simulink model "KerstingThreePhase"  (R2020a)
settings: Solver=ode45  StartTime=0.0  StopTime=2  RelTol=1e-3  EnableMultiTasking=on
undefined symbols (not defined in the file): Ac, Bc, Cc, Dc, j
libraries: powerlib x14, powerlib_meascontrol x9, simulink_extras x6
settings Model: Creator=Matus  LastModifiedBy=VaioPC
settings DataIOCC: LimitDataPoints=on  SaveFormat=Array  ReturnWorkspaceOutputs=off
settings OptimizationCC: LifeSpan=inf
settings DebuggingCC: UnderspecifiedInitializationDetection=Classic  MergeDetectMultiDrivingBlocksExec=none  StateNameClashWarn=warning  SFUnexpectedBacktrackingDiag=warning  SFNoUnconditionalDefaultTransitionDiag=warning  SFExecutionAtInitializationDiag=none  ArithmeticOperatorsInVariantConditions=warning
settings HardwareCC: ProdBitPerPointer=32  ProdBitPerSizeT=32  ProdBitPerPtrDiffT=32  ProdLargestAtomicFloat=None  ProdIntDivRoundTo=Undefined  ProdEndianess=Unspecified  ProdWordSize=32  ProdHWDeviceType=32-bit Generic
settings ModelReferenceCC: PropagateSignalLabelsOutOfModel=off
settings SFSimCC: SimUseLocalCustomCode=off  CustomCodeUndefinedFunction=UseInterfaceOnly
settings RTWCC: RTWUseLocalCustomCode=off
settings CodeAppCC: StateflowObjectComments=on
settings GRTTargetCC: TargetLangStandard=C89/C90 (ANSI)
settings ConfigComp: CovMetricSettings=dw  CovHtmlReporting=on  CovSaveCumulativeToWorkspaceVar=on  CovSaveSingleToWorkspaceVar=on  CovExternalEMLEnable=off
settings SimscapeCC: SimscapeNormalizeSystem=off

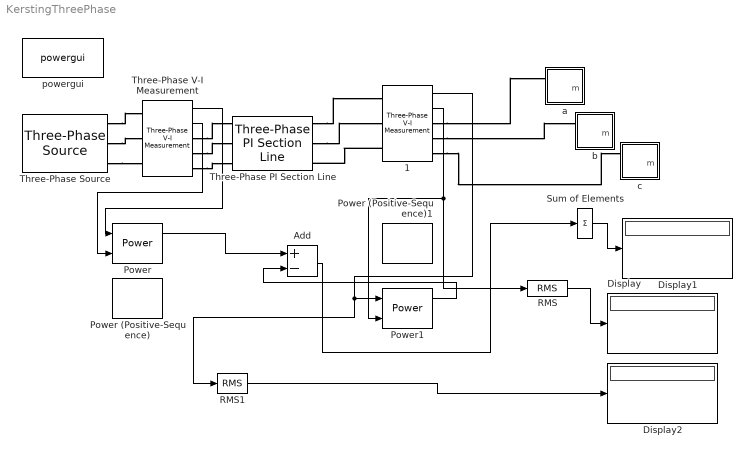
== system KerstingThreePhase ==
  1 : powerlib/Measurements/Three-Phase V-I Measurement  VoltageMeasurement=phase-to-ground  SetLabelV=off  LabelV=Vabc  Vpu=off  VpuLL=off  CurrentMeasurement=yes  SetLabelI=off  LabelI=Iabc  Ipu=off  Pbase=100e6  Vbase=500e3  OutputType=Complex  PhasorSimulation=off  PSBequivalent=0
  Add : Sum  Inputs=+-
  Display : Display
  Display1 : Display
  Display2 : Display
  Power : powerlib_meascontrol/Measurements/Power  Freq=60  Vinit=[1, 0]  Iinit=[1, 0]  Ts=0
  Power (Positive-Sequence) : powerlib_meascontrol/Measurements/Power (Positive-Sequence)  Freq=60  Vinit=[0, 0]  Iinit=[0, 0]  Ts=0
      settings: SourceProductBaseCode=PS
  Power (Positive-Sequence)1 : powerlib_meascontrol/Measurements/Power (Positive-Sequence)  Freq=60  Vinit=[0, 0]  Iinit=[0, 0]  Ts=0
      settings: SourceProductBaseCode=PS
  Power1 : powerlib_meascontrol/Measurements/Power  Freq=60  Vinit=[1, 0]  Iinit=[1, 0]  Ts=0
  RMS : powerlib_meascontrol/Measurements/RMS  TrueRMS=on  Freq=60  RMSInit=120  Ts=0
  RMS1 : powerlib_meascontrol/Measurements/RMS  TrueRMS=on  Freq=60  RMSInit=120  Ts=0
  Sum of Elements : Sum  Inputs=+
  Three-Phase PI Section Line : powerlib/Elements/Three-Phase PI Section Line  LConnTagsString=a|b|c  RConnTagsString=A|B|C  Frequency=60  Resistances=[ 0.1902 0.4807]  Inductances="[ 1.0336e-3  3.1935e-3]"  Capacitances=[12.74e-9 7.751e-9]  Length=1.8182
  Three-Phase V-I Measurement : powerlib/Measurements/Three-Phase V-I Measurement  VoltageMeasurement=phase-to-ground  SetLabelV=off  LabelV=Vabc  Vpu=off  VpuLL=off  CurrentMeasurement=yes  SetLabelI=off  LabelI=Iabc  Ipu=off  Pbase=100e6  Vbase=500e3  OutputType=Complex  PhasorSimulation=off  PSBequivalent=0
  Three-Phase Source : powerlib/Electrical Sources/Three-Phase Source  InternalConnection=Yg  VoltagePhases=off  Voltage=12470  PhaseAngle=0  Voltage_phases=[25e3 25e3 25e3]/sqrt(3)  PhaseAngles_phases=[0 -120 +120]  Frequency=60  NonIdealSource=on  SpecifyImpedance=on  Resistance=0.8929  Inductance=16.58e-3  ShortCircuitLevel=500e6  BaseVoltage=12470  XRratio=3  BusType=swing  Pref=0  Qref=0  Prefabc=[10e3, 10e3, 10e3]  Qrefabc=[0, 0, 0]  Qmin=-inf  Qmax=inf
  a : Subsystem  DialogController=POWERSYS.PowerSysDialog  mask(Single-Phase Dynamic Load){NominalVoltage=[ 7.1999e3 60 ], ActiveReactivePowers=[2.7e6 1.3077e6], PositiveSequence=[1 0], ExternalControl=off, NpNq=[0 0], TimeConstants=[0  0  0  0], MinimumVoltage=0.7, LoadFlowParameters=[4,0,0,0,0]}
      mask prompts: NominalVoltage "Nominal voltage and frequency  [Vn(Vrms) fn(Hz)]:"; ActiveReactivePowers "Active and reactive power at initial voltage [Po(W) Qo(var)]:"; PositiveSequence "Initial voltage Vo [Mag(pu) Phase (deg.)]:"; ExternalControl "External control of PQ"; NpNq "Parameters [ np  nq ]:"; TimeConstants "Time constants [Tp1 Tp2 Tq1 Tq2]  (s):"; MinimumVoltage "Minimum voltage Vmin (pu):"; LoadFlowParameters "Load Flow parameters"
      mask help:
      | Implements a single-phase dynamic load. Active  power P and reactive
      | power Q absorbed by the load vary as function of voltage V  according to the
      | following equations:
      |
      |   If V>Vmin, P and Q vary as follows:
      |        P = Po * (V/Vo)^np * (1+Tp1.s)/(1+Tp2.s)
      |        Q = Qo * (V/Vo)^nq * (1+Tq1.s)/(1+Tq2.s)
      |   if V<Vmin
      |      Same equations with np=nq=2 (constant impedance load)
      mask init:
      | block = gcb;
      | Ts = 50e-6;
      | %
      | Vnom=NominalVoltage(1); 
      | fnom=NominalVoltage(2);
      | P0=ActiveReactivePowers(1);
      | Q0=ActiveReactivePowers(2);
      | Mag_V0=PositiveSequence(1); 
      | Pha_V0=PositiveSequence(2);
      | V0_d=Mag_V0*cos(Pha_V0*pi/180);
      | V0_q=Mag_V0*sin(Pha_V0*pi/180);
      | np=NpNq(1);
      | nq=NpNq(2);
      | Tp1=TimeConstants(1); 
      | Tp2=TimeConstants(2); 
      | Tq1=TimeConstants(3); 
      | Tq2=TimeConstants(4);
      | Vbase=Vnom/sqrt(3)*sqrt(2);
      | % initial value of positive-sequence current I1
      | I1_init=(P0-j*Q0)/((V0_d-j*V0_q)*Vnom)/sqrt(3)*sqrt(2);
      | Mag_ia=abs(I1_init);
      | Phase_ia=angle(I1_init)*180/pi;
      | %
      | Vmin=MinimumVoltage;
      | PQext=ExternalControl;
      | a=exp(j*2*pi/3);
      | power_initmask();
      mask Help: helpview(psbhelp)
      mask Callback ExternalControl: powericon('ThreePhaseDynamicLoadCback',gcb);
      mask Display:
      | plot(-45,-45,45,45,[0,9,18,24,29,30,29,24,18,9,0,-9,-18,-24,-29,-30,-29,-24,-18,-9,0]*.9,[30,29,24,18,9,0,-9,-18,-24,-29,-30,-29,-24,-18,-9,0,9,18,24,29,30]*.9)
      | plot([0,0,10,0,-10,0]*1.1,[15,-5,-5,-15,-5,-5]*1.1)
  b : Subsystem  DialogController=POWERSYS.PowerSysDialog  mask(Single-Phase Dynamic Load){NominalVoltage=[ 7.1999e3 60 ], ActiveReactivePowers=[3.3250e6 1.0929e6], PositiveSequence=[1 0], ExternalControl=off, NpNq=[0 0], TimeConstants=[0  0  0  0], MinimumVoltage=0.7, LoadFlowParameters=[4,0,0,0,0]}
      mask prompts: NominalVoltage "Nominal voltage and frequency  [Vn(Vrms) fn(Hz)]:"; ActiveReactivePowers "Active and reactive power at initial voltage [Po(W) Qo(var)]:"; PositiveSequence "Initial voltage Vo [Mag(pu) Phase (deg.)]:"; ExternalControl "External control of PQ"; NpNq "Parameters [ np  nq ]:"; TimeConstants "Time constants [Tp1 Tp2 Tq1 Tq2]  (s):"; MinimumVoltage "Minimum voltage Vmin (pu):"; LoadFlowParameters "Load Flow parameters"
      mask help:
      | Implements a single-phase dynamic load. Active  power P and reactive
      | power Q absorbed by the load vary as function of voltage V  according to the
      | following equations:
      |
      |   If V>Vmin, P and Q vary as follows:
      |        P = Po * (V/Vo)^np * (1+Tp1.s)/(1+Tp2.s)
      |        Q = Qo * (V/Vo)^nq * (1+Tq1.s)/(1+Tq2.s)
      |   if V<Vmin
      |      Same equations with np=nq=2 (constant impedance load)
      mask init: same as KerstingThreePhase/a
      mask Help: helpview(psbhelp)
      mask Callback ExternalControl: powericon('ThreePhaseDynamicLoadCback',gcb);
      mask Display:
      | plot(-45,-45,45,45,[0,9,18,24,29,30,29,24,18,9,0,-9,-18,-24,-29,-30,-29,-24,-18,-9,0]*.9,[30,29,24,18,9,0,-9,-18,-24,-29,-30,-29,-24,-18,-9,0,9,18,24,29,30]*.9)
      | plot([0,0,10,0,-10,0]*1.1,[15,-5,-5,-15,-5,-5]*1.1)
  c : Subsystem  DialogController=POWERSYS.PowerSysDialog  mask(Single-Phase Dynamic Load){NominalVoltage=[ 7.1999e3 60 ], ActiveReactivePowers=[2.1250e6 1.3170e6], PositiveSequence=[1 0], ExternalControl=off, NpNq=[0 0], TimeConstants=[0  0  0  0], MinimumVoltage=0.7, LoadFlowParameters=[4,0,0,0,0]}
      mask prompts: NominalVoltage "Nominal voltage and frequency  [Vn(Vrms) fn(Hz)]:"; ActiveReactivePowers "Active and reactive power at initial voltage [Po(W) Qo(var)]:"; PositiveSequence "Initial voltage Vo [Mag(pu) Phase (deg.)]:"; ExternalControl "External control of PQ"; NpNq "Parameters [ np  nq ]:"; TimeConstants "Time constants [Tp1 Tp2 Tq1 Tq2]  (s):"; MinimumVoltage "Minimum voltage Vmin (pu):"; LoadFlowParameters "Load Flow parameters"
      mask help:
      | Implements a single-phase dynamic load. Active  power P and reactive
      | power Q absorbed by the load vary as function of voltage V  according to the
      | following equations:
      |
      |   If V>Vmin, P and Q vary as follows:
      |        P = Po * (V/Vo)^np * (1+Tp1.s)/(1+Tp2.s)
      |        Q = Qo * (V/Vo)^nq * (1+Tq1.s)/(1+Tq2.s)
      |   if V<Vmin
      |      Same equations with np=nq=2 (constant impedance load)
      mask init: same as KerstingThreePhase/a
      mask Help: helpview(psbhelp)
      mask Callback ExternalControl: powericon('ThreePhaseDynamicLoadCback',gcb);
      mask Display:
      | plot(-45,-45,45,45,[0,9,18,24,29,30,29,24,18,9,0,-9,-18,-24,-29,-30,-29,-24,-18,-9,0]*.9,[30,29,24,18,9,0,-9,-18,-24,-29,-30,-29,-24,-18,-9,0,9,18,24,29,30]*.9)
      | plot([0,0,10,0,-10,0]*1.1,[15,-5,-5,-15,-5,-5]*1.1)
  powergui : powerlib/powergui  Priority=1  SimulationMode=Discrete  SampleTime=50e-6  frequency=60  Iterations=50  frequencyindice=60  Pbase=100e6  ErrMax=1e-4  UnitsV=kV  UnitsW=MW  buscounter=0  FunctionMessages=off  echomessages=off  EnableUseOfTLC=off  CurrentSourceSwitches=off  DisableSnubberDevices=off  DisableRonSwitches=off  DisableVfSwitches=off  DisplayEquations=off  AutomaticDiscreteSolvers=off  SolverType=Tustin/Backward Euler (TBE)  Interpol=off  ExternalGateDelay=off  methode=off  Ts=100  x0status=blocks  SPID=on  SwTol=0  HookPort=off  NonlinearTolerance=1e-4  nMaxIteration=100  ContinueOnMaxIteration=off  RestoreLinks=warning  ResistiveCurrentMeasurement=off  Frange=[0:2:500]  Ylog=off  Xlog=on  ShowGrid=off  save=off  variable=ZData  structure=0  ZoomFFT=off  StartTime=0.0  cycles=1  DisplayStyle=1  fundamental=60  FreqAxis=off  MaxFrequency=1000  frequencyindicesteady=1  RmsSteady=2  display=off
  wires:
  Three-Phase V-I Measurement/2 -> Power/2
  Three-Phase V-I Measurement/1 -> Power/1
  1/1 -> Power1/1, RMS1/1
  1/2 -> Power1/2, RMS/1
  RMS/1 -> Display/1
  RMS1/1 -> Display2/1
  Add/1 -> Sum of Elements/1
  Power/1 -> Add/1
  Power1/1 -> Add/2
  Sum of Elements/1 -> Display1/1
  connections:
  Three-Phase Source/RConn1 -- Three-Phase V-I Measurement/LConn1
  Three-Phase Source/RConn2 -- Three-Phase V-I Measurement/LConn2
  Three-Phase Source/RConn3 -- Three-Phase V-I Measurement/LConn3
  1/LConn3 -- Three-Phase PI Section Line/RConn3
  Three-Phase PI Section Line/RConn2 -- 1/LConn2
  Three-Phase PI Section Line/RConn1 -- 1/LConn1
  Three-Phase V-I Measurement/RConn1 -- Three-Phase PI Section Line/LConn1
  Three-Phase V-I Measurement/RConn2 -- Three-Phase PI Section Line/LConn2
  Three-Phase V-I Measurement/RConn3 -- Three-Phase PI Section Line/LConn3
  1/RConn1 -- a/LConn1
  1/RConn2 -- b/LConn1
  1/RConn3 -- c/LConn1

== system KerstingThreePhase/a ==
  Controlled Current Source : powerlib/Electrical Sources/Controlled Current Source  Initialize=on  Source_Type=AC  Amplitude=0  Phase=0  Frequency=0  Measurements=None
  Gain : Gain  Gain=-1
  Ground1 : powerlib/Elements/Ground  LConnTagsString=a
  Measurement list : Subsystem
  PQ : Ground
  Voltage Measurement1 : powerlib/Measurements/Voltage Measurement  PhasorSimulation=off  OutputType=Complex  PSBequivalent=0
  model : Subsystem
  a : PMIOPort  Tag=PMCPort  Side=Left
  b : PMIOPort  Tag=PMCPort  Port=2  Side=Left
  m : Outport  InitialOutput=[0,0,0]  VectorParamsAs1DForOutWhenUnconnected=off
  wires:
  Gain/1 -> Controlled Current Source/1
  Measurement list/1(Out1) -> m/1
  model/1(i) -> Gain/1
  Voltage Measurement1/1 -> model/1(v)
  PQ/1 -> model/2(PQ)
  model/2(m) -> Measurement list/1(In1)
  connections:
  Controlled Current Source/LConn1 -- Ground1/LConn1 -- b/RConn1 -- Voltage Measurement1/LConn2
  Controlled Current Source/RConn1 -- a/RConn1 -- Voltage Measurement1/LConn1

== system KerstingThreePhase/b ==
  Controlled Current Source : powerlib/Electrical Sources/Controlled Current Source  Initialize=on  Source_Type=AC  Amplitude=0  Phase=0  Frequency=0  Measurements=None
  Gain : Gain  Gain=-1
  Ground1 : powerlib/Elements/Ground  LConnTagsString=a
  Measurement list : Subsystem
  PQ : Ground
  Voltage Measurement1 : powerlib/Measurements/Voltage Measurement  PhasorSimulation=off  OutputType=Complex  PSBequivalent=0
  model : Subsystem
  a : PMIOPort  Tag=PMCPort  Side=Left
  b : PMIOPort  Tag=PMCPort  Port=2  Side=Left
  m : Outport  InitialOutput=[0,0,0]  VectorParamsAs1DForOutWhenUnconnected=off
  wires:
  Gain/1 -> Controlled Current Source/1
  Measurement list/1(Out1) -> m/1
  model/1(i) -> Gain/1
  Voltage Measurement1/1 -> model/1(v)
  PQ/1 -> model/2(PQ)
  model/2(m) -> Measurement list/1(In1)
  connections:
  Controlled Current Source/LConn1 -- Voltage Measurement1/LConn2 -- Ground1/LConn1 -- b/RConn1
  Controlled Current Source/RConn1 -- a/RConn1 -- Voltage Measurement1/LConn1

== system KerstingThreePhase/c ==
  Controlled Current Source : powerlib/Electrical Sources/Controlled Current Source  Initialize=on  Source_Type=AC  Amplitude=0  Phase=0  Frequency=0  Measurements=None
  Gain : Gain  Gain=-1
  Ground1 : powerlib/Elements/Ground  LConnTagsString=a
  Measurement list : Subsystem
  PQ : Ground
  Voltage Measurement1 : powerlib/Measurements/Voltage Measurement  PhasorSimulation=off  OutputType=Complex  PSBequivalent=0
  model : Subsystem
  a : PMIOPort  Tag=PMCPort  Side=Left
  b : PMIOPort  Tag=PMCPort  Port=2  Side=Left
  m : Outport  InitialOutput=[0,0,0]  VectorParamsAs1DForOutWhenUnconnected=off
  wires:
  Gain/1 -> Controlled Current Source/1
  Measurement list/1(Out1) -> m/1
  model/1(i) -> Gain/1
  Voltage Measurement1/1 -> model/1(v)
  PQ/1 -> model/2(PQ)
  model/2(m) -> Measurement list/1(In1)
  connections:
  Controlled Current Source/LConn1 -- Voltage Measurement1/LConn2 -- Ground1/LConn1 -- b/RConn1
  Controlled Current Source/RConn1 -- a/RConn1 -- Voltage Measurement1/LConn1

== system KerstingThreePhase/a/Measurement list ==
  In1 : Inport
  Bus Creator1 : BusCreator  Inputs=3
  Demux : Demux  Outputs=[1,1,1]
  Out1 : Outport  VectorParamsAs1DForOutWhenUnconnected=off
  wires:
  In1/1 -> Demux/1
  Bus Creator1/1 -> Out1/1
  Demux/2 -> Bus Creator1/2  "Active power P (W)"
  Demux/1 -> Bus Creator1/1  "Positive-sequence voltage V (pu)"
  Demux/3 -> Bus Creator1/3  "Reactive power Q (var)"

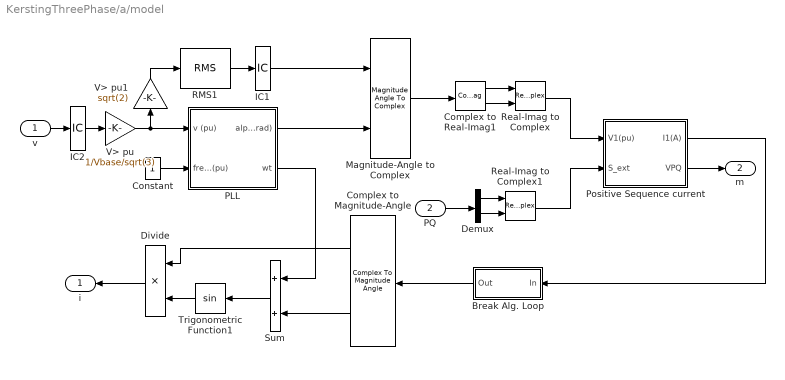
== system KerstingThreePhase/a/model ==
  v : Inport
  PQ : Inport  Port=2
  Break Alg. Loop : Subsystem
  Complex to Magnitude-Angle : ComplexToMagnitudeAngle
  Complex to Real-Imag1 : ComplexToRealImag
  Constant : Constant
  Demux : Demux  Outputs=2
      settings: DisplayOption=none
  Divide : Product  Inputs=**
  IC1 : InitialCondition
  IC2 : InitialCondition
  Magnitude-Angle to Complex : MagnitudeAngleToComplex
  PLL : Subsystem  mask{freq=fnom}
      mask prompts: freq "Initial frequency (Hz)"
  Positive Sequence current : Subsystem
  RMS1 : powerlib_meascontrol/Measurements/RMS  TrueRMS=on  Freq=fnom  RMSInit=1  Ts=0
  Real-Imag to Complex : RealImagToComplex
  Real-Imag to Complex1 : RealImagToComplex
  Sum : Sum
  Trigonometric Function1 : Trigonometry
  V> pu : Gain  Gain=1/Vbase/sqrt(3)  SaturateOnIntegerOverflow=on  OutDataTypeStr=Inherit: Same as input  ParamDataTypeStr=Inherit: Same as input
  V> pu1 : Gain  Gain=sqrt(2)  SaturateOnIntegerOverflow=on  OutDataTypeStr=Inherit: Same as input  ParamDataTypeStr=Inherit: Same as input
  i : Outport  VectorParamsAs1DForOutWhenUnconnected=off
  m : Outport  Port=2  VectorParamsAs1DForOutWhenUnconnected=off
  wires:
  IC2/1 -> V> pu/1
  V> pu1/1 -> RMS1/1
  IC1/1 -> Magnitude-Angle to Complex/1
  RMS1/1 -> IC1/1
  Break Alg. Loop/1(Out) -> Complex to Magnitude-Angle/1
  Divide/1 -> i/1
  Complex to Magnitude-Angle/1 -> Divide/1
  Trigonometric Function1/1 -> Divide/2
  Sum/1 -> Trigonometric Function1/1
  PLL/2(wt) -> Sum/1
  Complex to Magnitude-Angle/2 -> Sum/2
  PLL/1(alpha (rad)) -> Magnitude-Angle to Complex/2
  Constant/1 -> PLL/2(freq (pu))
  Magnitude-Angle to Complex/1 -> Complex to Real-Imag1/1
  Complex to Real-Imag1/2 -> Real-Imag to Complex/2
  Complex to Real-Imag1/1 -> Real-Imag to Complex/1
  v/1 -> IC2/1
  Positive Sequence current/2(VPQ) -> m/1
  Real-Imag to Complex1/1 -> Positive Sequence current/2(S_ext)
  Demux/2 -> Real-Imag to Complex1/2
  Demux/1 -> Real-Imag to Complex1/1
  PQ/1 -> Demux/1
  Positive Sequence current/1(I1(A)) -> Break Alg. Loop/1(In)
  Real-Imag to Complex/1 -> Positive Sequence current/1(V1(pu))
  V> pu/1 -> V> pu1/1, PLL/1(v (pu))

== system KerstingThreePhase/b/Measurement list ==
  In1 : Inport
  Bus Creator1 : BusCreator  Inputs=3
  Demux : Demux  Outputs=[1,1,1]
  Out1 : Outport  VectorParamsAs1DForOutWhenUnconnected=off
  wires:
  In1/1 -> Demux/1
  Bus Creator1/1 -> Out1/1
  Demux/2 -> Bus Creator1/2  "Active power P (W)"
  Demux/1 -> Bus Creator1/1  "Positive-sequence voltage V (pu)"
  Demux/3 -> Bus Creator1/3  "Reactive power Q (var)"

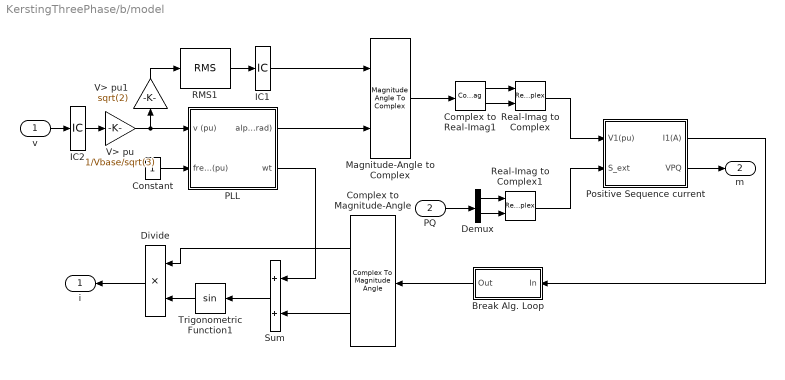
== system KerstingThreePhase/b/model ==
  v : Inport
  PQ : Inport  Port=2
  Break Alg. Loop : Subsystem
  Complex to Magnitude-Angle : ComplexToMagnitudeAngle
  Complex to Real-Imag1 : ComplexToRealImag
  Constant : Constant
  Demux : Demux  Outputs=2
      settings: DisplayOption=none
  Divide : Product  Inputs=**
  IC1 : InitialCondition
  IC2 : InitialCondition
  Magnitude-Angle to Complex : MagnitudeAngleToComplex
  PLL : Subsystem  mask{freq=fnom}
      mask prompts: freq "Initial frequency (Hz)"
  Positive Sequence current : Subsystem
  RMS1 : powerlib_meascontrol/Measurements/RMS  TrueRMS=on  Freq=fnom  RMSInit=1  Ts=0
  Real-Imag to Complex : RealImagToComplex
  Real-Imag to Complex1 : RealImagToComplex
  Sum : Sum
  Trigonometric Function1 : Trigonometry
  V> pu : Gain  Gain=1/Vbase/sqrt(3)  SaturateOnIntegerOverflow=on  OutDataTypeStr=Inherit: Same as input  ParamDataTypeStr=Inherit: Same as input
  V> pu1 : Gain  Gain=sqrt(2)  SaturateOnIntegerOverflow=on  OutDataTypeStr=Inherit: Same as input  ParamDataTypeStr=Inherit: Same as input
  i : Outport  VectorParamsAs1DForOutWhenUnconnected=off
  m : Outport  Port=2  VectorParamsAs1DForOutWhenUnconnected=off
  wires:
  IC2/1 -> V> pu/1
  V> pu1/1 -> RMS1/1
  IC1/1 -> Magnitude-Angle to Complex/1
  RMS1/1 -> IC1/1
  Break Alg. Loop/1(Out) -> Complex to Magnitude-Angle/1
  Divide/1 -> i/1
  Complex to Magnitude-Angle/1 -> Divide/1
  Trigonometric Function1/1 -> Divide/2
  Sum/1 -> Trigonometric Function1/1
  PLL/2(wt) -> Sum/1
  Complex to Magnitude-Angle/2 -> Sum/2
  PLL/1(alpha (rad)) -> Magnitude-Angle to Complex/2
  Constant/1 -> PLL/2(freq (pu))
  Magnitude-Angle to Complex/1 -> Complex to Real-Imag1/1
  Complex to Real-Imag1/2 -> Real-Imag to Complex/2
  Complex to Real-Imag1/1 -> Real-Imag to Complex/1
  v/1 -> IC2/1
  Positive Sequence current/2(VPQ) -> m/1
  Real-Imag to Complex1/1 -> Positive Sequence current/2(S_ext)
  Demux/2 -> Real-Imag to Complex1/2
  Demux/1 -> Real-Imag to Complex1/1
  PQ/1 -> Demux/1
  Positive Sequence current/1(I1(A)) -> Break Alg. Loop/1(In)
  Real-Imag to Complex/1 -> Positive Sequence current/1(V1(pu))
  V> pu/1 -> V> pu1/1, PLL/1(v (pu))

== system KerstingThreePhase/c/Measurement list ==
  In1 : Inport
  Bus Creator1 : BusCreator  Inputs=3
  Demux : Demux  Outputs=[1,1,1]
  Out1 : Outport  VectorParamsAs1DForOutWhenUnconnected=off
  wires:
  In1/1 -> Demux/1
  Bus Creator1/1 -> Out1/1
  Demux/2 -> Bus Creator1/2  "Active power P (W)"
  Demux/1 -> Bus Creator1/1  "Positive-sequence voltage V (pu)"
  Demux/3 -> Bus Creator1/3  "Reactive power Q (var)"

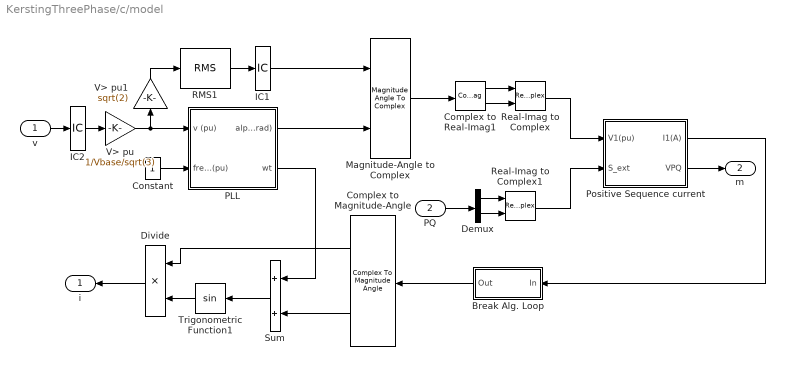
== system KerstingThreePhase/c/model ==
  v : Inport
  PQ : Inport  Port=2
  Break Alg. Loop : Subsystem
  Complex to Magnitude-Angle : ComplexToMagnitudeAngle
  Complex to Real-Imag1 : ComplexToRealImag
  Constant : Constant
  Demux : Demux  Outputs=2
      settings: DisplayOption=none
  Divide : Product  Inputs=**
  IC1 : InitialCondition
  IC2 : InitialCondition
  Magnitude-Angle to Complex : MagnitudeAngleToComplex
  PLL : Subsystem  mask{freq=fnom}
      mask prompts: freq "Initial frequency (Hz)"
  Positive Sequence current : Subsystem
  RMS1 : powerlib_meascontrol/Measurements/RMS  TrueRMS=on  Freq=fnom  RMSInit=1  Ts=0
  Real-Imag to Complex : RealImagToComplex
  Real-Imag to Complex1 : RealImagToComplex
  Sum : Sum
  Trigonometric Function1 : Trigonometry
  V> pu : Gain  Gain=1/Vbase/sqrt(3)  SaturateOnIntegerOverflow=on  OutDataTypeStr=Inherit: Same as input  ParamDataTypeStr=Inherit: Same as input
  V> pu1 : Gain  Gain=sqrt(2)  SaturateOnIntegerOverflow=on  OutDataTypeStr=Inherit: Same as input  ParamDataTypeStr=Inherit: Same as input
  i : Outport  VectorParamsAs1DForOutWhenUnconnected=off
  m : Outport  Port=2  VectorParamsAs1DForOutWhenUnconnected=off
  wires:
  IC2/1 -> V> pu/1
  V> pu1/1 -> RMS1/1
  IC1/1 -> Magnitude-Angle to Complex/1
  RMS1/1 -> IC1/1
  Break Alg. Loop/1(Out) -> Complex to Magnitude-Angle/1
  Divide/1 -> i/1
  Complex to Magnitude-Angle/1 -> Divide/1
  Trigonometric Function1/1 -> Divide/2
  Sum/1 -> Trigonometric Function1/1
  PLL/2(wt) -> Sum/1
  Complex to Magnitude-Angle/2 -> Sum/2
  PLL/1(alpha (rad)) -> Magnitude-Angle to Complex/2
  Constant/1 -> PLL/2(freq (pu))
  Magnitude-Angle to Complex/1 -> Complex to Real-Imag1/1
  Complex to Real-Imag1/2 -> Real-Imag to Complex/2
  Complex to Real-Imag1/1 -> Real-Imag to Complex/1
  v/1 -> IC2/1
  Positive Sequence current/2(VPQ) -> m/1
  Real-Imag to Complex1/1 -> Positive Sequence current/2(S_ext)
  Demux/2 -> Real-Imag to Complex1/2
  Demux/1 -> Real-Imag to Complex1/1
  PQ/1 -> Demux/1
  Positive Sequence current/1(I1(A)) -> Break Alg. Loop/1(In)
  Real-Imag to Complex/1 -> Positive Sequence current/1(V1(pu))
  V> pu/1 -> V> pu1/1, PLL/1(v (pu))

== system KerstingThreePhase/a/model/Break Alg. Loop ==
  In : Inport
  Complex to Real-Imag : ComplexToRealImag
  Real-Imag to Complex : RealImagToComplex
  imag : simulink_extras/Additional Linear/Transfer Fcn (with initial outputs)  N=[1]  D="[100e-6  1]"  Y0=imag(I1_init*exp(-j*Pha_V0*pi/180))  U0=imag(I1_init*exp(-j*Pha_V0*pi/180))
  real : simulink_extras/Additional Linear/Transfer Fcn (with initial outputs)  N=[1]  D="[100e-6  1]"  Y0=real(I1_init*exp(-j*Pha_V0*pi/180))  U0=real(I1_init*exp(-j*Pha_V0*pi/180))
  Out : Outport  VectorParamsAs1DForOutWhenUnconnected=off
  wires:
  In/1 -> Complex to Real-Imag/1
  Real-Imag to Complex/1 -> Out/1
  Complex to Real-Imag/1 -> real/1
  real/1 -> Real-Imag to Complex/1
  Complex to Real-Imag/2 -> imag/1
  imag/1 -> Real-Imag to Complex/2

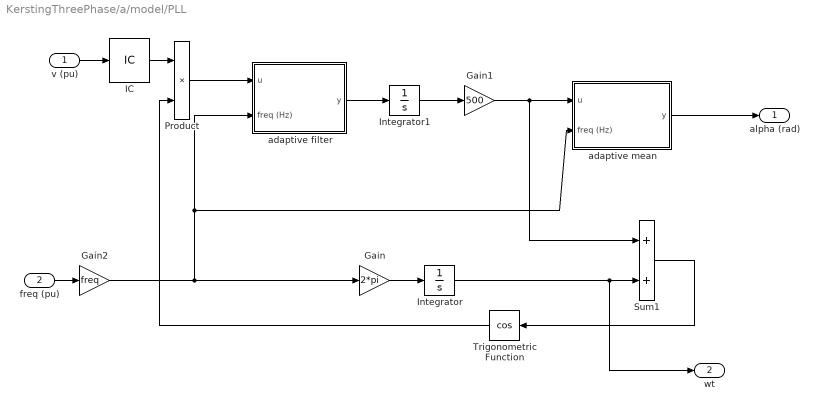
== system KerstingThreePhase/a/model/PLL ==
  v (pu) : Inport
  freq (pu) : Inport  Port=2
  Gain : Gain  Gain=2*pi
  Gain1 : Gain  Gain=500
  Gain2 : Gain  Gain=freq
  IC : InitialCondition
  Integrator : Integrator
  Integrator1 : Integrator
  Product : Product  Inputs=**  RndMeth=Zero
  Sum1 : Sum  InputSameDT=on  SaturateOnIntegerOverflow=on  OutDataTypeStr=Inherit: Same as first input
  Trigonometric Function : Trigonometry  Operator=cos
  adaptive filter : Subsystem
  adaptive mean : Subsystem
  alpha (rad) : Outport  VectorParamsAs1DForOutWhenUnconnected=off
  wt : Outport  Port=2  VectorParamsAs1DForOutWhenUnconnected=off
  wires:
  IC/1 -> Product/1
  v (pu)/1 -> IC/1
  Product/1 -> adaptive filter/1(u)
  adaptive filter/1(y) -> Integrator1/1
  Gain/1 -> Integrator/1
  Integrator/1 -> wt/1, Sum1/2
  Sum1/1 -> Trigonometric Function/1
  Gain1/1 -> adaptive mean/1(u), Sum1/1
  Integrator1/1 -> Gain1/1
  adaptive mean/1(y) -> alpha (rad)/1
  Trigonometric Function/1 -> Product/2
  Gain2/1 -> Gain/1, adaptive mean/2(freq (Hz)), adaptive filter/2(freq (Hz))
  freq (pu)/1 -> Gain2/1

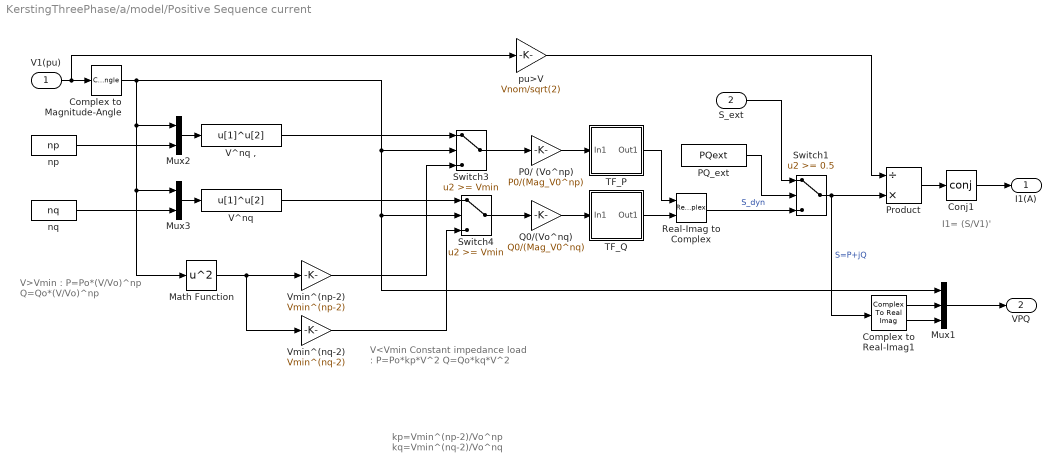
== system KerstingThreePhase/a/model/Positive Sequence current ==
  note: I1= (S/V1)'
  note: V>Vmin :
      |
      |    P=Po*(V/Vo)^np
      |    Q=Qo*(V/Vo)^np
  note: V<Vmin
      | Constant impedance load :
      |
      |  P=Po*kp*V^2
      | Q=Qo*kq*V^2
  note: kp=Vmin^(np-2)/Vo^np
      | kq=Vmin^(nq-2)/Vo^nq
  V1(pu) : Inport
  S_ext : Inport  Port=2
  Complex to Magnitude-Angle : ComplexToMagnitudeAngle  Output=Magnitude
  Complex to Real-Imag1 : ComplexToRealImag
  Conj1 : Math  Operator=conj  SignedPower=on  SaturateOnIntegerOverflow=on
  Math Function : Math  Operator=square  SignedPower=on  SaturateOnIntegerOverflow=on
  Mux1 : Mux  Inputs=3
  Mux2 : Mux  Inputs=2
  Mux3 : Mux  Inputs=2
  P0/ (Vo^np) : Gain  Gain=P0/(Mag_V0^np)  SaturateOnIntegerOverflow=on  OutDataTypeStr=Inherit: Same as input  ParamDataTypeStr=Inherit: Same as input
  PQ_ext : Constant  Value=PQext
  Product : Product  Inputs=/*  InputSameDT=on  SaturateOnIntegerOverflow=on  OutDataTypeStr=Inherit: Same as first input
  Q0/(Vo^nq) : Gain  Gain=Q0/(Mag_V0^nq)  SaturateOnIntegerOverflow=on  OutDataTypeStr=Inherit: Same as input  ParamDataTypeStr=Inherit: Same as input
  Real-Imag to Complex : RealImagToComplex
  Switch1 : Switch  Threshold=0.5  InputSameDT=on
  Switch3 : Switch  Threshold=Vmin  InputSameDT=on
  Switch4 : Switch  Threshold=Vmin  InputSameDT=on
  TF_P : Subsystem  mask(Transfer function){T1=Tp1, T2=Tp2, V_Init=P0}
      mask prompts: T1 "Time constant T1 (s):"; T2 "Time constant T2 (s):"; V_Init "Initial input and output :"
      mask help:
      | This block implements a continuous transfer function:
      |
      |          1+T1s
      | H(s)= ------
      |          1+T2s
      |
      | States are initialized according to  initial input and output value so that simulation starts in steady state.
      mask init:
      | numc=[T1 1];
      | denc=[T2 1];
      | [Ac,Bc,Cc,Dc]=tf2ss(numc,denc);
      | 
      | % Compute Initial states
      | I=eye(size(Ac));
      | x0c=inv(-Ac)*Bc*V_Init;
      mask Display: disp('1+T1s\n---\n1+T2s')
  TF_Q : Subsystem  mask(Transfer function){T1=Tq1, T2=Tq2, V_Init=Q0}
      mask prompts: T1 "Time constant T1 (s):"; T2 "Time constant T2 (s):"; V_Init "Initial input and output :"
      mask help:
      | This block implements a continuous transfer function:
      |
      |          1+T1s
      | H(s)= ------
      |          1+T2s
      |
      | States are initialized according to  initial input and output value so that simulation starts in steady state.
      mask init:
      | numc=[T1 1];
      | denc=[T2 1];
      | [Ac,Bc,Cc,Dc]=tf2ss(numc,denc);
      | 
      | % Compute Initial states
      | I=eye(size(Ac));
      | x0c=inv(-Ac)*Bc*V_Init;
      mask Display: disp('1+T1s\n---\n1+T2s')
  V^nq : Fcn  Expr=u[1]^u[2]
  V^nq , : Fcn  Expr=u[1]^u[2]
  Vmin^(np-2) : Gain  Gain=Vmin^(np-2)  SaturateOnIntegerOverflow=on  OutDataTypeStr=Inherit: Same as input  ParamDataTypeStr=Inherit: Same as input
  Vmin^(nq-2) : Gain  Gain=Vmin^(nq-2)  SaturateOnIntegerOverflow=on  OutDataTypeStr=Inherit: Same as input  ParamDataTypeStr=Inherit: Same as input
  np : Constant  Value=np
  nq : Constant  Value=nq
  pu>V : Gain  Gain=Vnom/sqrt(2)  SaturateOnIntegerOverflow=on  OutDataTypeStr=Inherit: Same as input  ParamDataTypeStr=Inherit: Same as input
  I1(A) : Outport  VectorParamsAs1DForOutWhenUnconnected=off
  VPQ : Outport  Port=2  VectorParamsAs1DForOutWhenUnconnected=off
  wires:
  TF_Q/1(Out1) -> Real-Imag to Complex/2
  TF_P/1(Out1) -> Real-Imag to Complex/1
  Complex to Real-Imag1/2 -> Mux1/3
  Complex to Real-Imag1/1 -> Mux1/2
  Mux1/1 -> VPQ/1
  Complex to Magnitude-Angle/1 -> Mux1/1, Switch4/2, Switch3/2, Mux2/1, Mux3/1, Math Function/1
  pu>V/1 -> Product/1
  PQ_ext/1 -> Switch1/2
  S_ext/1 -> Switch1/1
  Real-Imag to Complex/1 -> Switch1/3  "S_dyn"
  Switch1/1 -> Complex to Real-Imag1/1, Product/2  "S=P+jQ"
  Conj1/1 -> I1(A)/1
  Product/1 -> Conj1/1
  Switch4/1 -> Q0/(Vo^nq)/1
  P0/ (Vo^np)/1 -> TF_P/1(In1)
  Q0/(Vo^nq)/1 -> TF_Q/1(In1)
  Switch3/1 -> P0/ (Vo^np)/1
  np/1 -> Mux2/2
  Mux2/1 -> V^nq ,/1
  nq/1 -> Mux3/2
  Mux3/1 -> V^nq/1
  V1(pu)/1 -> pu>V/1, Complex to Magnitude-Angle/1
  V^nq/1 -> Switch4/1
  Math Function/1 -> Vmin^(np-2)/1, Vmin^(nq-2)/1
  Vmin^(np-2)/1 -> Switch3/3
  V^nq ,/1 -> Switch3/1
  Vmin^(nq-2)/1 -> Switch4/3

== system KerstingThreePhase/b/model/Break Alg. Loop ==
  In : Inport
  Complex to Real-Imag : ComplexToRealImag
  Real-Imag to Complex : RealImagToComplex
  imag : simulink_extras/Additional Linear/Transfer Fcn (with initial outputs)  N=[1]  D="[100e-6  1]"  Y0=imag(I1_init*exp(-j*Pha_V0*pi/180))  U0=imag(I1_init*exp(-j*Pha_V0*pi/180))
  real : simulink_extras/Additional Linear/Transfer Fcn (with initial outputs)  N=[1]  D="[100e-6  1]"  Y0=real(I1_init*exp(-j*Pha_V0*pi/180))  U0=real(I1_init*exp(-j*Pha_V0*pi/180))
  Out : Outport  VectorParamsAs1DForOutWhenUnconnected=off
  wires:
  In/1 -> Complex to Real-Imag/1
  Real-Imag to Complex/1 -> Out/1
  Complex to Real-Imag/1 -> real/1
  real/1 -> Real-Imag to Complex/1
  Complex to Real-Imag/2 -> imag/1
  imag/1 -> Real-Imag to Complex/2

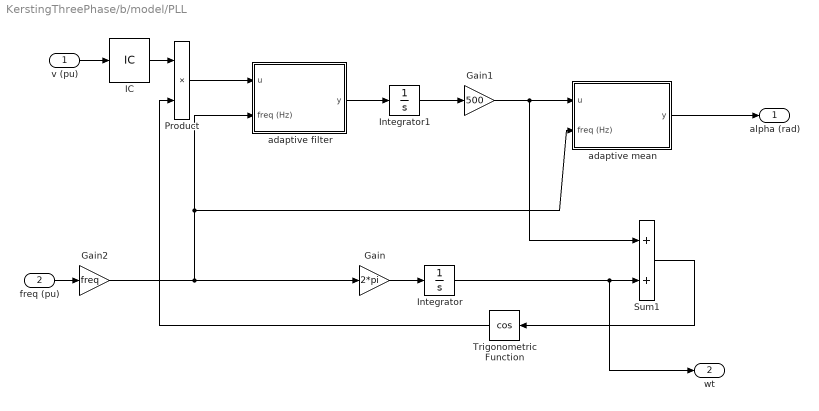
== system KerstingThreePhase/b/model/PLL ==
  v (pu) : Inport
  freq (pu) : Inport  Port=2
  Gain : Gain  Gain=2*pi
  Gain1 : Gain  Gain=500
  Gain2 : Gain  Gain=freq
  IC : InitialCondition
  Integrator : Integrator
  Integrator1 : Integrator
  Product : Product  Inputs=**  RndMeth=Zero
  Sum1 : Sum  InputSameDT=on  SaturateOnIntegerOverflow=on  OutDataTypeStr=Inherit: Same as first input
  Trigonometric Function : Trigonometry  Operator=cos
  adaptive filter : Subsystem
  adaptive mean : Subsystem
  alpha (rad) : Outport  VectorParamsAs1DForOutWhenUnconnected=off
  wt : Outport  Port=2  VectorParamsAs1DForOutWhenUnconnected=off
  wires:
  IC/1 -> Product/1
  v (pu)/1 -> IC/1
  Product/1 -> adaptive filter/1(u)
  adaptive filter/1(y) -> Integrator1/1
  Gain/1 -> Integrator/1
  Integrator/1 -> wt/1, Sum1/2
  Sum1/1 -> Trigonometric Function/1
  Gain1/1 -> adaptive mean/1(u), Sum1/1
  Integrator1/1 -> Gain1/1
  adaptive mean/1(y) -> alpha (rad)/1
  Trigonometric Function/1 -> Product/2
  Gain2/1 -> Gain/1, adaptive mean/2(freq (Hz)), adaptive filter/2(freq (Hz))
  freq (pu)/1 -> Gain2/1

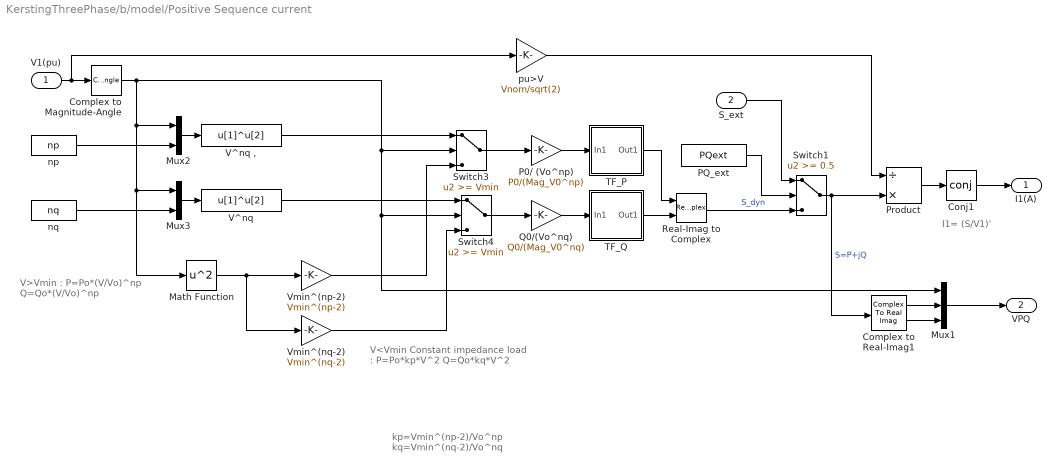
== system KerstingThreePhase/b/model/Positive Sequence current ==
  note: I1= (S/V1)'
  note: V>Vmin :
      |
      |    P=Po*(V/Vo)^np
      |    Q=Qo*(V/Vo)^np
  note: V<Vmin
      | Constant impedance load :
      |
      |  P=Po*kp*V^2
      | Q=Qo*kq*V^2
  note: kp=Vmin^(np-2)/Vo^np
      | kq=Vmin^(nq-2)/Vo^nq
  V1(pu) : Inport
  S_ext : Inport  Port=2
  Complex to Magnitude-Angle : ComplexToMagnitudeAngle  Output=Magnitude
  Complex to Real-Imag1 : ComplexToRealImag
  Conj1 : Math  Operator=conj  SignedPower=on  SaturateOnIntegerOverflow=on
  Math Function : Math  Operator=square  SignedPower=on  SaturateOnIntegerOverflow=on
  Mux1 : Mux  Inputs=3
  Mux2 : Mux  Inputs=2
  Mux3 : Mux  Inputs=2
  P0/ (Vo^np) : Gain  Gain=P0/(Mag_V0^np)  SaturateOnIntegerOverflow=on  OutDataTypeStr=Inherit: Same as input  ParamDataTypeStr=Inherit: Same as input
  PQ_ext : Constant  Value=PQext
  Product : Product  Inputs=/*  InputSameDT=on  SaturateOnIntegerOverflow=on  OutDataTypeStr=Inherit: Same as first input
  Q0/(Vo^nq) : Gain  Gain=Q0/(Mag_V0^nq)  SaturateOnIntegerOverflow=on  OutDataTypeStr=Inherit: Same as input  ParamDataTypeStr=Inherit: Same as input
  Real-Imag to Complex : RealImagToComplex
  Switch1 : Switch  Threshold=0.5  InputSameDT=on
  Switch3 : Switch  Threshold=Vmin  InputSameDT=on
  Switch4 : Switch  Threshold=Vmin  InputSameDT=on
  TF_P : Subsystem  mask(Transfer function){T1=Tp1, T2=Tp2, V_Init=P0}
      mask prompts: T1 "Time constant T1 (s):"; T2 "Time constant T2 (s):"; V_Init "Initial input and output :"
      mask help:
      | This block implements a continuous transfer function:
      |
      |          1+T1s
      | H(s)= ------
      |          1+T2s
      |
      | States are initialized according to  initial input and output value so that simulation starts in steady state.
      mask init:
      | numc=[T1 1];
      | denc=[T2 1];
      | [Ac,Bc,Cc,Dc]=tf2ss(numc,denc);
      | 
      | % Compute Initial states
      | I=eye(size(Ac));
      | x0c=inv(-Ac)*Bc*V_Init;
      mask Display: disp('1+T1s\n---\n1+T2s')
  TF_Q : Subsystem  mask(Transfer function){T1=Tq1, T2=Tq2, V_Init=Q0}
      mask prompts: T1 "Time constant T1 (s):"; T2 "Time constant T2 (s):"; V_Init "Initial input and output :"
      mask help:
      | This block implements a continuous transfer function:
      |
      |          1+T1s
      | H(s)= ------
      |          1+T2s
      |
      | States are initialized according to  initial input and output value so that simulation starts in steady state.
      mask init:
      | numc=[T1 1];
      | denc=[T2 1];
      | [Ac,Bc,Cc,Dc]=tf2ss(numc,denc);
      | 
      | % Compute Initial states
      | I=eye(size(Ac));
      | x0c=inv(-Ac)*Bc*V_Init;
      mask Display: disp('1+T1s\n---\n1+T2s')
  V^nq : Fcn  Expr=u[1]^u[2]
  V^nq , : Fcn  Expr=u[1]^u[2]
  Vmin^(np-2) : Gain  Gain=Vmin^(np-2)  SaturateOnIntegerOverflow=on  OutDataTypeStr=Inherit: Same as input  ParamDataTypeStr=Inherit: Same as input
  Vmin^(nq-2) : Gain  Gain=Vmin^(nq-2)  SaturateOnIntegerOverflow=on  OutDataTypeStr=Inherit: Same as input  ParamDataTypeStr=Inherit: Same as input
  np : Constant  Value=np
  nq : Constant  Value=nq
  pu>V : Gain  Gain=Vnom/sqrt(2)  SaturateOnIntegerOverflow=on  OutDataTypeStr=Inherit: Same as input  ParamDataTypeStr=Inherit: Same as input
  I1(A) : Outport  VectorParamsAs1DForOutWhenUnconnected=off
  VPQ : Outport  Port=2  VectorParamsAs1DForOutWhenUnconnected=off
  wires:
  TF_Q/1(Out1) -> Real-Imag to Complex/2
  TF_P/1(Out1) -> Real-Imag to Complex/1
  Complex to Real-Imag1/2 -> Mux1/3
  Complex to Real-Imag1/1 -> Mux1/2
  Mux1/1 -> VPQ/1
  Complex to Magnitude-Angle/1 -> Mux1/1, Switch4/2, Switch3/2, Mux2/1, Mux3/1, Math Function/1
  pu>V/1 -> Product/1
  PQ_ext/1 -> Switch1/2
  S_ext/1 -> Switch1/1
  Real-Imag to Complex/1 -> Switch1/3  "S_dyn"
  Switch1/1 -> Complex to Real-Imag1/1, Product/2  "S=P+jQ"
  Conj1/1 -> I1(A)/1
  Product/1 -> Conj1/1
  Switch4/1 -> Q0/(Vo^nq)/1
  P0/ (Vo^np)/1 -> TF_P/1(In1)
  Q0/(Vo^nq)/1 -> TF_Q/1(In1)
  Switch3/1 -> P0/ (Vo^np)/1
  np/1 -> Mux2/2
  Mux2/1 -> V^nq ,/1
  nq/1 -> Mux3/2
  Mux3/1 -> V^nq/1
  V1(pu)/1 -> pu>V/1, Complex to Magnitude-Angle/1
  V^nq/1 -> Switch4/1
  Math Function/1 -> Vmin^(np-2)/1, Vmin^(nq-2)/1
  Vmin^(np-2)/1 -> Switch3/3
  V^nq ,/1 -> Switch3/1
  Vmin^(nq-2)/1 -> Switch4/3

== system KerstingThreePhase/c/model/Break Alg. Loop ==
  In : Inport
  Complex to Real-Imag : ComplexToRealImag
  Real-Imag to Complex : RealImagToComplex
  imag : simulink_extras/Additional Linear/Transfer Fcn (with initial outputs)  N=[1]  D="[100e-6  1]"  Y0=imag(I1_init*exp(-j*Pha_V0*pi/180))  U0=imag(I1_init*exp(-j*Pha_V0*pi/180))
  real : simulink_extras/Additional Linear/Transfer Fcn (with initial outputs)  N=[1]  D="[100e-6  1]"  Y0=real(I1_init*exp(-j*Pha_V0*pi/180))  U0=real(I1_init*exp(-j*Pha_V0*pi/180))
  Out : Outport  VectorParamsAs1DForOutWhenUnconnected=off
  wires:
  In/1 -> Complex to Real-Imag/1
  Real-Imag to Complex/1 -> Out/1
  Complex to Real-Imag/1 -> real/1
  real/1 -> Real-Imag to Complex/1
  Complex to Real-Imag/2 -> imag/1
  imag/1 -> Real-Imag to Complex/2

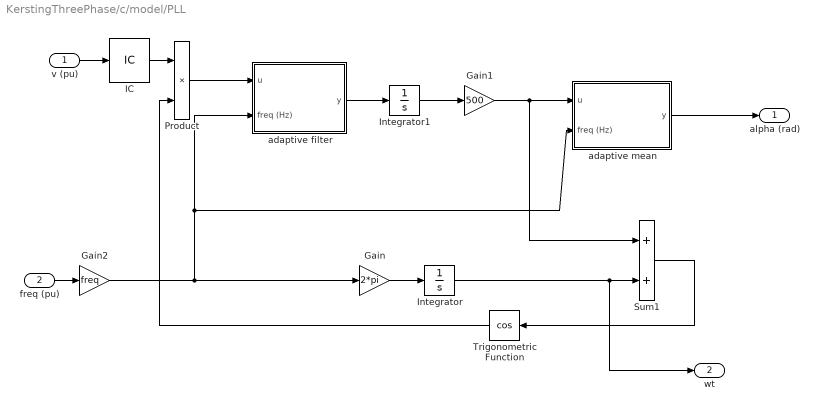
== system KerstingThreePhase/c/model/PLL ==
  v (pu) : Inport
  freq (pu) : Inport  Port=2
  Gain : Gain  Gain=2*pi
  Gain1 : Gain  Gain=500
  Gain2 : Gain  Gain=freq
  IC : InitialCondition
  Integrator : Integrator
  Integrator1 : Integrator
  Product : Product  Inputs=**  RndMeth=Zero
  Sum1 : Sum  InputSameDT=on  SaturateOnIntegerOverflow=on  OutDataTypeStr=Inherit: Same as first input
  Trigonometric Function : Trigonometry  Operator=cos
  adaptive filter : Subsystem
  adaptive mean : Subsystem
  alpha (rad) : Outport  VectorParamsAs1DForOutWhenUnconnected=off
  wt : Outport  Port=2  VectorParamsAs1DForOutWhenUnconnected=off
  wires:
  IC/1 -> Product/1
  v (pu)/1 -> IC/1
  Product/1 -> adaptive filter/1(u)
  adaptive filter/1(y) -> Integrator1/1
  Gain/1 -> Integrator/1
  Integrator/1 -> wt/1, Sum1/2
  Sum1/1 -> Trigonometric Function/1
  Gain1/1 -> adaptive mean/1(u), Sum1/1
  Integrator1/1 -> Gain1/1
  adaptive mean/1(y) -> alpha (rad)/1
  Trigonometric Function/1 -> Product/2
  Gain2/1 -> Gain/1, adaptive mean/2(freq (Hz)), adaptive filter/2(freq (Hz))
  freq (pu)/1 -> Gain2/1

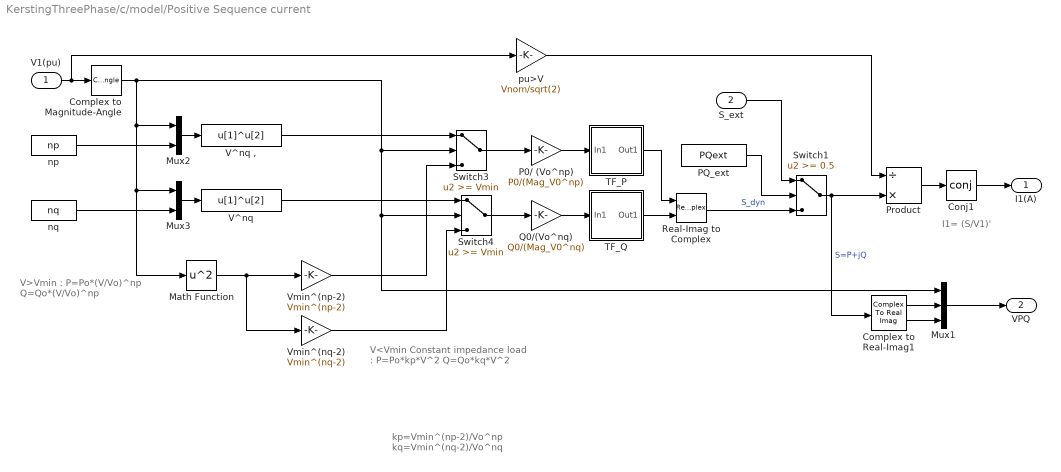
== system KerstingThreePhase/c/model/Positive Sequence current ==
  note: I1= (S/V1)'
  note: V>Vmin :
      |
      |    P=Po*(V/Vo)^np
      |    Q=Qo*(V/Vo)^np
  note: V<Vmin
      | Constant impedance load :
      |
      |  P=Po*kp*V^2
      | Q=Qo*kq*V^2
  note: kp=Vmin^(np-2)/Vo^np
      | kq=Vmin^(nq-2)/Vo^nq
  V1(pu) : Inport
  S_ext : Inport  Port=2
  Complex to Magnitude-Angle : ComplexToMagnitudeAngle  Output=Magnitude
  Complex to Real-Imag1 : ComplexToRealImag
  Conj1 : Math  Operator=conj  SignedPower=on  SaturateOnIntegerOverflow=on
  Math Function : Math  Operator=square  SignedPower=on  SaturateOnIntegerOverflow=on
  Mux1 : Mux  Inputs=3
  Mux2 : Mux  Inputs=2
  Mux3 : Mux  Inputs=2
  P0/ (Vo^np) : Gain  Gain=P0/(Mag_V0^np)  SaturateOnIntegerOverflow=on  OutDataTypeStr=Inherit: Same as input  ParamDataTypeStr=Inherit: Same as input
  PQ_ext : Constant  Value=PQext
  Product : Product  Inputs=/*  InputSameDT=on  SaturateOnIntegerOverflow=on  OutDataTypeStr=Inherit: Same as first input
  Q0/(Vo^nq) : Gain  Gain=Q0/(Mag_V0^nq)  SaturateOnIntegerOverflow=on  OutDataTypeStr=Inherit: Same as input  ParamDataTypeStr=Inherit: Same as input
  Real-Imag to Complex : RealImagToComplex
  Switch1 : Switch  Threshold=0.5  InputSameDT=on
  Switch3 : Switch  Threshold=Vmin  InputSameDT=on
  Switch4 : Switch  Threshold=Vmin  InputSameDT=on
  TF_P : Subsystem  mask(Transfer function){T1=Tp1, T2=Tp2, V_Init=P0}
      mask prompts: T1 "Time constant T1 (s):"; T2 "Time constant T2 (s):"; V_Init "Initial input and output :"
      mask help:
      | This block implements a continuous transfer function:
      |
      |          1+T1s
      | H(s)= ------
      |          1+T2s
      |
      | States are initialized according to  initial input and output value so that simulation starts in steady state.
      mask init:
      | numc=[T1 1];
      | denc=[T2 1];
      | [Ac,Bc,Cc,Dc]=tf2ss(numc,denc);
      | 
      | % Compute Initial states
      | I=eye(size(Ac));
      | x0c=inv(-Ac)*Bc*V_Init;
      mask Display: disp('1+T1s\n---\n1+T2s')
  TF_Q : Subsystem  mask(Transfer function){T1=Tq1, T2=Tq2, V_Init=Q0}
      mask prompts: T1 "Time constant T1 (s):"; T2 "Time constant T2 (s):"; V_Init "Initial input and output :"
      mask help:
      | This block implements a continuous transfer function:
      |
      |          1+T1s
      | H(s)= ------
      |          1+T2s
      |
      | States are initialized according to  initial input and output value so that simulation starts in steady state.
      mask init:
      | numc=[T1 1];
      | denc=[T2 1];
      | [Ac,Bc,Cc,Dc]=tf2ss(numc,denc);
      | 
      | % Compute Initial states
      | I=eye(size(Ac));
      | x0c=inv(-Ac)*Bc*V_Init;
      mask Display: disp('1+T1s\n---\n1+T2s')
  V^nq : Fcn  Expr=u[1]^u[2]
  V^nq , : Fcn  Expr=u[1]^u[2]
  Vmin^(np-2) : Gain  Gain=Vmin^(np-2)  SaturateOnIntegerOverflow=on  OutDataTypeStr=Inherit: Same as input  ParamDataTypeStr=Inherit: Same as input
  Vmin^(nq-2) : Gain  Gain=Vmin^(nq-2)  SaturateOnIntegerOverflow=on  OutDataTypeStr=Inherit: Same as input  ParamDataTypeStr=Inherit: Same as input
  np : Constant  Value=np
  nq : Constant  Value=nq
  pu>V : Gain  Gain=Vnom/sqrt(2)  SaturateOnIntegerOverflow=on  OutDataTypeStr=Inherit: Same as input  ParamDataTypeStr=Inherit: Same as input
  I1(A) : Outport  VectorParamsAs1DForOutWhenUnconnected=off
  VPQ : Outport  Port=2  VectorParamsAs1DForOutWhenUnconnected=off
  wires:
  TF_Q/1(Out1) -> Real-Imag to Complex/2
  TF_P/1(Out1) -> Real-Imag to Complex/1
  Complex to Real-Imag1/2 -> Mux1/3
  Complex to Real-Imag1/1 -> Mux1/2
  Mux1/1 -> VPQ/1
  Complex to Magnitude-Angle/1 -> Mux1/1, Switch4/2, Switch3/2, Mux2/1, Mux3/1, Math Function/1
  pu>V/1 -> Product/1
  PQ_ext/1 -> Switch1/2
  S_ext/1 -> Switch1/1
  Real-Imag to Complex/1 -> Switch1/3  "S_dyn"
  Switch1/1 -> Complex to Real-Imag1/1, Product/2  "S=P+jQ"
  Conj1/1 -> I1(A)/1
  Product/1 -> Conj1/1
  Switch4/1 -> Q0/(Vo^nq)/1
  P0/ (Vo^np)/1 -> TF_P/1(In1)
  Q0/(Vo^nq)/1 -> TF_Q/1(In1)
  Switch3/1 -> P0/ (Vo^np)/1
  np/1 -> Mux2/2
  Mux2/1 -> V^nq ,/1
  nq/1 -> Mux3/2
  Mux3/1 -> V^nq/1
  V1(pu)/1 -> pu>V/1, Complex to Magnitude-Angle/1
  V^nq/1 -> Switch4/1
  Math Function/1 -> Vmin^(np-2)/1, Vmin^(nq-2)/1
  Vmin^(np-2)/1 -> Switch3/3
  V^nq ,/1 -> Switch3/1
  Vmin^(nq-2)/1 -> Switch4/3

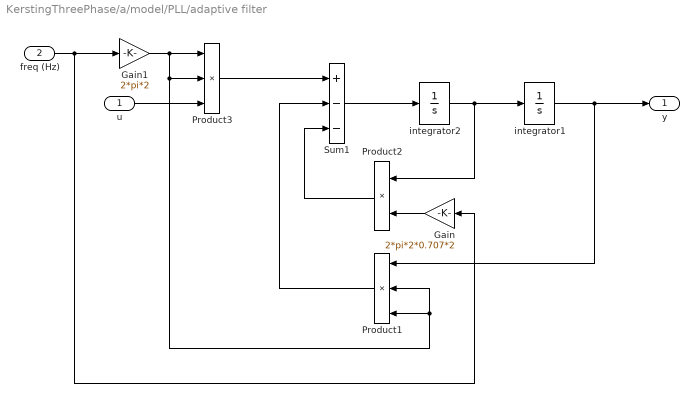
== system KerstingThreePhase/a/model/PLL/adaptive filter ==
  u : Inport
  freq (Hz) : Inport  Port=2
  Gain : Gain  Gain=2*pi*2*0.707*2
  Gain1 : Gain  Gain=2*pi*2
  Product1 : Product  Inputs=***  RndMeth=Zero
  Product2 : Product  Inputs=**  RndMeth=Zero
  Product3 : Product  Inputs=***  RndMeth=Zero
  Sum1 : Sum  Inputs=+--  InputSameDT=on  SaturateOnIntegerOverflow=on  OutDataTypeStr=Inherit: Same as first input
  integrator1 : Integrator
  integrator2 : Integrator
  y : Outport  VectorParamsAs1DForOutWhenUnconnected=off
  wires:
  integrator2/1 -> integrator1/1, Product2/1
  Sum1/1 -> integrator2/1
  Product2/1 -> Sum1/3
  Gain/1 -> Product2/2
  integrator1/1 -> y/1, Product1/1
  Product3/1 -> Sum1/1
  Gain1/1 -> Product3/1, Product3/2, Product1/2, Product1/3
  freq (Hz)/1 -> Gain1/1, Gain/1
  u/1 -> Product3/3
  Product1/1 -> Sum1/2

== system KerstingThreePhase/a/model/PLL/adaptive mean ==
  u : Inport
  freq (Hz) : Inport  Port=2
  Fcn : Fcn  Expr=u(1)+1e-6
  Math Function : Math  Operator=reciprocal  SignedPower=on  SaturateOnIntegerOverflow=on
  Product1 : Product  Inputs=**  RndMeth=Zero
  Sum : Sum  Inputs=+-  InputSameDT=on  SaturateOnIntegerOverflow=on  OutDataTypeStr=Inherit: Same as first input
  Variable Transport Delay : VariableTransportDelay  MaximumDelay=1/40  MaximumPoints=4096
  integrator : Integrator
  y : Outport  VectorParamsAs1DForOutWhenUnconnected=off
  wires:
  Fcn/1 -> Product1/2, Math Function/1
  freq (Hz)/1 -> Fcn/1
  Math Function/1 -> Variable Transport Delay/2
  Variable Transport Delay/1 -> Sum/2
  integrator/1 -> Sum/1, Variable Transport Delay/1
  Sum/1 -> Product1/1
  u/1 -> integrator/1
  Product1/1 -> y/1

== system KerstingThreePhase/a/model/Positive Sequence current/TF_P ==
  In1 : Inport
  State-Space : StateSpace  A=Ac  B=Bc  C=Cc  D=Dc  InitialCondition=x0c
  Out1 : Outport  VectorParamsAs1DForOutWhenUnconnected=off
  wires:
  In1/1 -> State-Space/1
  State-Space/1 -> Out1/1

== system KerstingThreePhase/a/model/Positive Sequence current/TF_Q ==
  In1 : Inport
  State-Space : StateSpace  A=Ac  B=Bc  C=Cc  D=Dc  InitialCondition=x0c
  Out1 : Outport  VectorParamsAs1DForOutWhenUnconnected=off
  wires:
  State-Space/1 -> Out1/1
  In1/1 -> State-Space/1

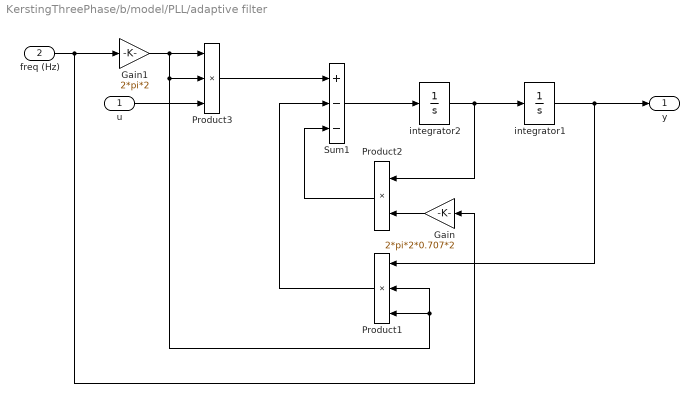
== system KerstingThreePhase/b/model/PLL/adaptive filter ==
  u : Inport
  freq (Hz) : Inport  Port=2
  Gain : Gain  Gain=2*pi*2*0.707*2
  Gain1 : Gain  Gain=2*pi*2
  Product1 : Product  Inputs=***  RndMeth=Zero
  Product2 : Product  Inputs=**  RndMeth=Zero
  Product3 : Product  Inputs=***  RndMeth=Zero
  Sum1 : Sum  Inputs=+--  InputSameDT=on  SaturateOnIntegerOverflow=on  OutDataTypeStr=Inherit: Same as first input
  integrator1 : Integrator
  integrator2 : Integrator
  y : Outport  VectorParamsAs1DForOutWhenUnconnected=off
  wires:
  integrator2/1 -> integrator1/1, Product2/1
  Sum1/1 -> integrator2/1
  Product2/1 -> Sum1/3
  Gain/1 -> Product2/2
  integrator1/1 -> y/1, Product1/1
  Product3/1 -> Sum1/1
  Gain1/1 -> Product3/1, Product3/2, Product1/2, Product1/3
  freq (Hz)/1 -> Gain1/1, Gain/1
  u/1 -> Product3/3
  Product1/1 -> Sum1/2

== system KerstingThreePhase/b/model/PLL/adaptive mean ==
  u : Inport
  freq (Hz) : Inport  Port=2
  Fcn : Fcn  Expr=u(1)+1e-6
  Math Function : Math  Operator=reciprocal  SignedPower=on  SaturateOnIntegerOverflow=on
  Product1 : Product  Inputs=**  RndMeth=Zero
  Sum : Sum  Inputs=+-  InputSameDT=on  SaturateOnIntegerOverflow=on  OutDataTypeStr=Inherit: Same as first input
  Variable Transport Delay : VariableTransportDelay  MaximumDelay=1/40  MaximumPoints=4096
  integrator : Integrator
  y : Outport  VectorParamsAs1DForOutWhenUnconnected=off
  wires:
  Fcn/1 -> Product1/2, Math Function/1
  freq (Hz)/1 -> Fcn/1
  Math Function/1 -> Variable Transport Delay/2
  Variable Transport Delay/1 -> Sum/2
  integrator/1 -> Sum/1, Variable Transport Delay/1
  Sum/1 -> Product1/1
  u/1 -> integrator/1
  Product1/1 -> y/1

== system KerstingThreePhase/b/model/Positive Sequence current/TF_P ==
  In1 : Inport
  State-Space : StateSpace  A=Ac  B=Bc  C=Cc  D=Dc  InitialCondition=x0c
  Out1 : Outport  VectorParamsAs1DForOutWhenUnconnected=off
  wires:
  In1/1 -> State-Space/1
  State-Space/1 -> Out1/1

== system KerstingThreePhase/b/model/Positive Sequence current/TF_Q ==
  In1 : Inport
  State-Space : StateSpace  A=Ac  B=Bc  C=Cc  D=Dc  InitialCondition=x0c
  Out1 : Outport  VectorParamsAs1DForOutWhenUnconnected=off
  wires:
  State-Space/1 -> Out1/1
  In1/1 -> State-Space/1

== system KerstingThreePhase/c/model/PLL/adaptive filter ==
  u : Inport
  freq (Hz) : Inport  Port=2
  Gain : Gain  Gain=2*pi*2*0.707*2
  Gain1 : Gain  Gain=2*pi*2
  Product1 : Product  Inputs=***  RndMeth=Zero
  Product2 : Product  Inputs=**  RndMeth=Zero
  Product3 : Product  Inputs=***  RndMeth=Zero
  Sum1 : Sum  Inputs=+--  InputSameDT=on  SaturateOnIntegerOverflow=on  OutDataTypeStr=Inherit: Same as first input
  integrator1 : Integrator
  integrator2 : Integrator
  y : Outport  VectorParamsAs1DForOutWhenUnconnected=off
  wires:
  integrator2/1 -> integrator1/1, Product2/1
  Sum1/1 -> integrator2/1
  Product2/1 -> Sum1/3
  Gain/1 -> Product2/2
  integrator1/1 -> y/1, Product1/1
  Product3/1 -> Sum1/1
  Gain1/1 -> Product3/1, Product3/2, Product1/2, Product1/3
  freq (Hz)/1 -> Gain1/1, Gain/1
  u/1 -> Product3/3
  Product1/1 -> Sum1/2

== system KerstingThreePhase/c/model/PLL/adaptive mean ==
  u : Inport
  freq (Hz) : Inport  Port=2
  Fcn : Fcn  Expr=u(1)+1e-6
  Math Function : Math  Operator=reciprocal  SignedPower=on  SaturateOnIntegerOverflow=on
  Product1 : Product  Inputs=**  RndMeth=Zero
  Sum : Sum  Inputs=+-  InputSameDT=on  SaturateOnIntegerOverflow=on  OutDataTypeStr=Inherit: Same as first input
  Variable Transport Delay : VariableTransportDelay  MaximumDelay=1/40  MaximumPoints=4096
  integrator : Integrator
  y : Outport  VectorParamsAs1DForOutWhenUnconnected=off
  wires:
  Fcn/1 -> Product1/2, Math Function/1
  freq (Hz)/1 -> Fcn/1
  Math Function/1 -> Variable Transport Delay/2
  Variable Transport Delay/1 -> Sum/2
  integrator/1 -> Sum/1, Variable Transport Delay/1
  Sum/1 -> Product1/1
  u/1 -> integrator/1
  Product1/1 -> y/1

== system KerstingThreePhase/c/model/Positive Sequence current/TF_P ==
  In1 : Inport
  State-Space : StateSpace  A=Ac  B=Bc  C=Cc  D=Dc  InitialCondition=x0c
  Out1 : Outport  VectorParamsAs1DForOutWhenUnconnected=off
  wires:
  In1/1 -> State-Space/1
  State-Space/1 -> Out1/1

== system KerstingThreePhase/c/model/Positive Sequence current/TF_Q ==
  In1 : Inport
  State-Space : StateSpace  A=Ac  B=Bc  C=Cc  D=Dc  InitialCondition=x0c
  Out1 : Outport  VectorParamsAs1DForOutWhenUnconnected=off
  wires:
  State-Space/1 -> Out1/1
  In1/1 -> State-Space/1
